simulink model "exercise01"  (R2022a)
settings: Solver=VariableStepAuto  StartTime=0.0  StopTime=10  RelTol=1e-3
settings Model: Creator=cunis  LastModifiedBy=cunis

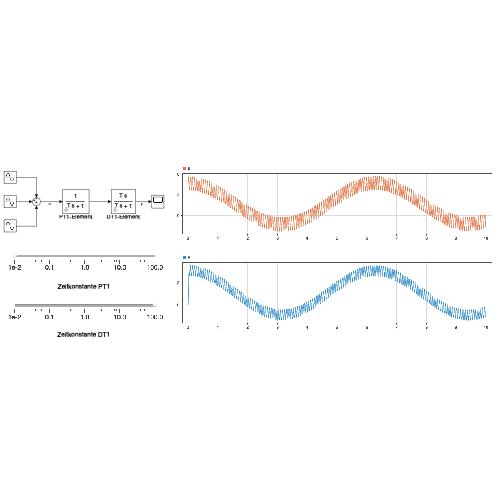
[thumbnail: Simulink's stored preview of the top-level diagram]
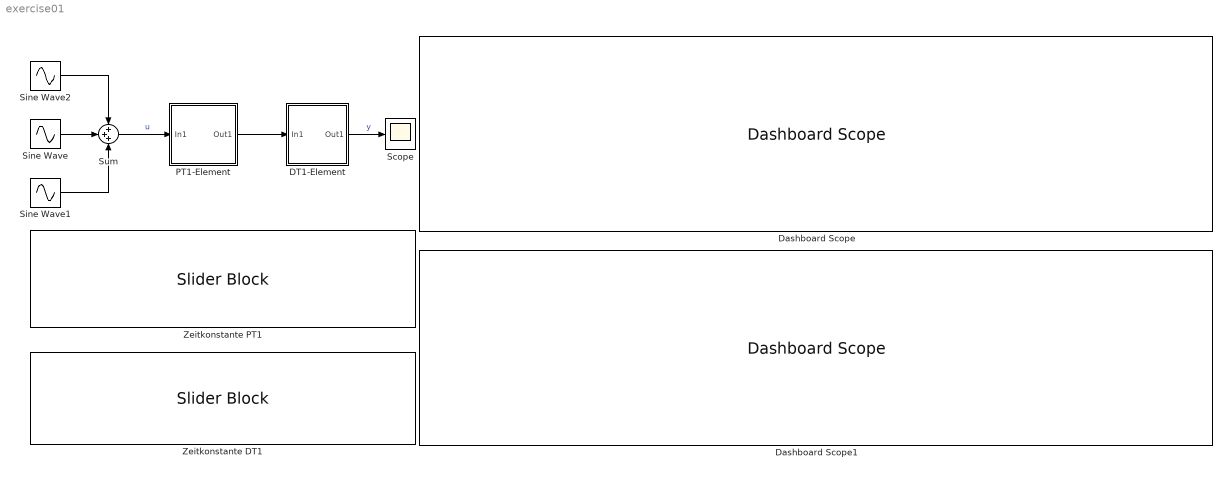
== system exercise01 ==
  DT1-Element : Subsystem
      mask Display: disp('T s\n----------\nT s + 1')
  Dashboard Scope : DashboardScope
  Dashboard Scope1 : DashboardScope
  PT1-Element : Subsystem
      mask Display: disp('1\n----------\nT s + 1')
  Scope : Scope
  Sine Wave : Sin  Amplitude=2  Frequency=0.01  Phase=1  SampleTime=0
  Sine Wave1 : Sin  Amplitude=3  Phase=pi/2  SampleTime=0
  Sine Wave2 : Sin  Frequency=100  SampleTime=0
  Sum : Sum  Inputs=+++
  Zeitkonstante DT1 : SliderBlock  LabelPosition=Hide  ScaleMin=0.01  ScaleType=Log
  Zeitkonstante PT1 : SliderBlock  LabelPosition=Hide  ScaleMin=0.01  ScaleType=Log
  wires:
  Sine Wave/1 -> Sum/2
  Sine Wave1/1 -> Sum/3
  Sine Wave2/1 -> Sum/1
  Sum/1 -> PT1-Element/1(In1)  "u"
  PT1-Element/1(Out1) -> DT1-Element/1(In1)
  DT1-Element/1(Out1) -> Scope/1  "y"

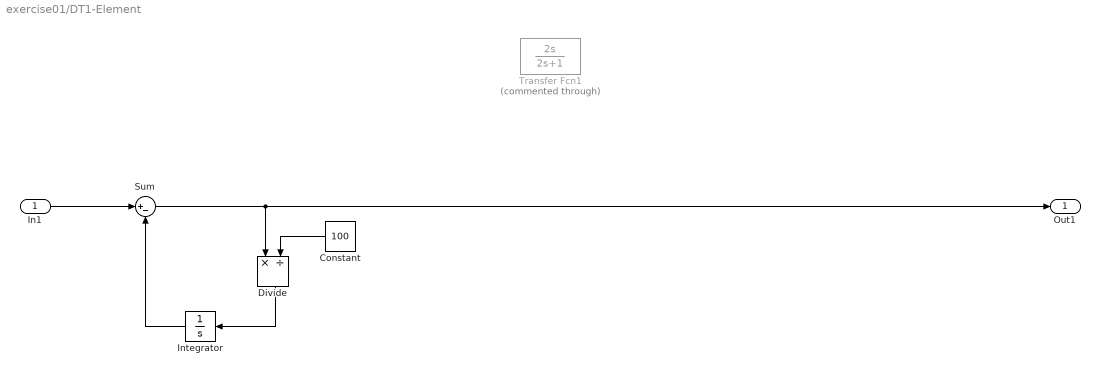
== system exercise01/DT1-Element ==
  In1 : Inport
  Constant : Constant  Value=100
  Divide : Product  Inputs=*/
  Integrator : Integrator
  Sum : Sum  Inputs=|+-
  Transfer Fcn1 : TransferFcn  Commented=through  Numerator=[2 0]  Denominator=[2 1]
  Out1 : Outport
  wires:
  In1/1 -> Sum/1
  Sum/1 -> Divide/1, Out1/1
  Integrator/1 -> Sum/2
  Divide/1 -> Integrator/1
  Constant/1 -> Divide/2

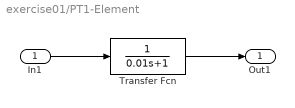
== system exercise01/PT1-Element ==
  In1 : Inport
  Transfer Fcn : TransferFcn  Denominator=[0.01,1]
  Out1 : Outport
  wires:
  Transfer Fcn/1 -> Out1/1
  In1/1 -> Transfer Fcn/1
